simulink library "sensorsLib"  (R2020b)
settings: Solver=VariableStepAuto  StartTime=0.0  StopTime=10.0  RelTol=1e-3
settings Model: Creator=dbell44  LastModifiedBy=dbell44

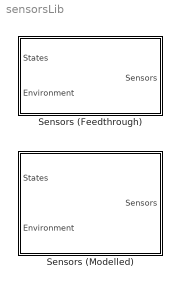
== system sensorsLib ==
  Sensors (Feedthrough) : Subsystem
  Sensors (Modelled) : Subsystem

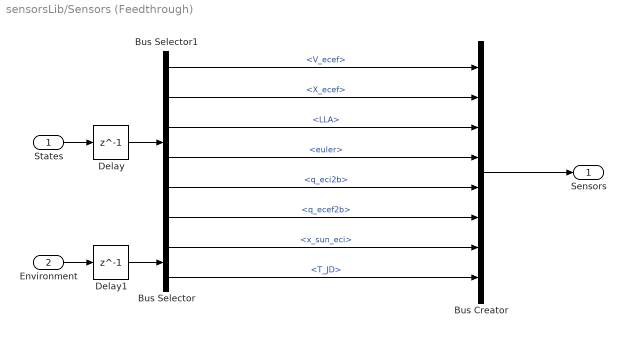
== system sensorsLib/Sensors (Feedthrough) ==
  States : Inport  OutDataTypeStr=Bus: States
  Environment : Inport  Port=2
  Bus Creator : BusCreator  Inputs=8
  Bus Selector : BusSelector  OutputSignals=x_sun_eci,T_JD
  Bus Selector1 : BusSelector  OutputSignals=V_ecef,X_ecef,LLA,euler,q_eci2b,q_ecef2b
  Delay : Delay  DelayLength=1  InitialCondition=0
  Delay1 : Delay  DelayLength=1  InitialCondition=0
  Sensors : Outport
  wires:
  Environment/1 -> Delay1/1
  Bus Selector/1 -> Bus Creator/7  "<x_sun_eci>"
  Bus Selector/2 -> Bus Creator/8  "<T_JD>"
  States/1 -> Delay/1
  Bus Creator/1 -> Sensors/1
  Bus Selector1/1 -> Bus Creator/1  "<V_ecef>"
  Bus Selector1/2 -> Bus Creator/2  "<X_ecef>"
  Bus Selector1/3 -> Bus Creator/3  "<LLA>"
  Bus Selector1/4 -> Bus Creator/4  "<euler>"
  Bus Selector1/5 -> Bus Creator/5  "<q_eci2b>"
  Bus Selector1/6 -> Bus Creator/6  "<q_ecef2b>"
  Delay/1 -> Bus Selector1/1
  Delay1/1 -> Bus Selector/1

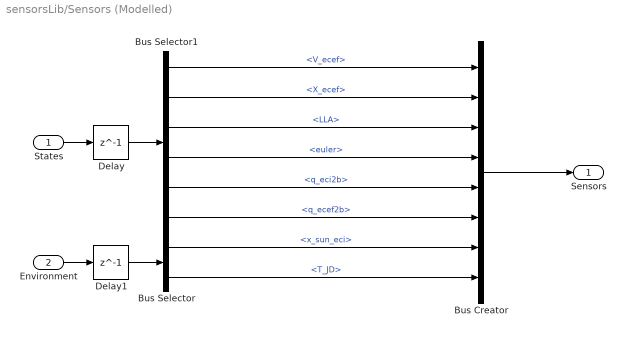
== system sensorsLib/Sensors (Modelled) ==
  States : Inport  OutDataTypeStr=Bus: States
  Environment : Inport  Port=2
  Bus Creator : BusCreator  Inputs=8
  Bus Selector : BusSelector  OutputSignals=x_sun_eci,T_JD
  Bus Selector1 : BusSelector  OutputSignals=V_ecef,X_ecef,LLA,euler,q_eci2b,q_ecef2b
  Delay : Delay  DelayLength=1  InitialCondition=0
  Delay1 : Delay  DelayLength=1  InitialCondition=0
  Sensors : Outport
  wires:
  Environment/1 -> Delay1/1
  Bus Selector/1 -> Bus Creator/7  "<x_sun_eci>"
  Bus Selector/2 -> Bus Creator/8  "<T_JD>"
  States/1 -> Delay/1
  Bus Creator/1 -> Sensors/1
  Bus Selector1/1 -> Bus Creator/1  "<V_ecef>"
  Bus Selector1/2 -> Bus Creator/2  "<X_ecef>"
  Bus Selector1/3 -> Bus Creator/3  "<LLA>"
  Bus Selector1/4 -> Bus Creator/4  "<euler>"
  Bus Selector1/5 -> Bus Creator/5  "<q_eci2b>"
  Bus Selector1/6 -> Bus Creator/6  "<q_ecef2b>"
  Delay/1 -> Bus Selector1/1
  Delay1/1 -> Bus Selector/1
